simulink model "unicycle_nonlinear_Cl"  (R2024a)
settings: Solver=VariableStepAuto  StartTime=0.0  StopTime=30  RelTol=1e-3
values from neighbouring files (symbols this model uses):
  AK = AK2 - BK/(eye(p_y)-D22*DK)*D22*CK    [report_controller_output_feedback_Hinf.m]    (also in report_controller_output_feedback_LMI.m = A+L_gain*C2+B2*K_gain; report_controller_state_feedback_H2.m = zeros(n,n); report_controller_state_feedback_Hinf.m = zeros(n,n))
  BK = BK2*(eye(p_y)-D22*DK)    [report_controller_output_feedback_Hinf.m]    (also in report_controller_output_feedback_LMI.m = -L_gain; report_controller_state_feedback_H2.m = zeros(n,p_y); report_controller_state_feedback_Hinf.m = zeros(n,p_y))
  C2 = [1 0 0 0 ... (first row only)    [report_controller_output_feedback_Hinf.m]    (also in report_controller_output_feedback_LMI.m; report_controller_state_feedback_H2.m; report_controller_state_feedback_Hinf.m; report_model_negative_theta.m)
  CK = (eye(m)-DK*D22)*CK2    [report_controller_output_feedback_Hinf.m]    (also in report_controller_output_feedback_LMI.m = K_gain; report_controller_state_feedback_H2.m = zeros(m,n); report_controller_state_feedback_Hinf.m = zeros(m,n))
  DK = (eye(m)+DK2*D22)\DK2    [report_controller_output_feedback_Hinf.m]    (also in report_controller_output_feedback_LMI.m = zeros(m,p_y); report_controller_state_feedback_H2.m = K_gain; report_controller_state_feedback_Hinf.m = K_gain)
  equilibrium = asin((M_w+M_p)*R_w/(M_p*L)*sin(theta))-theta    [report_model_equilibrium.m]    (also in report_model_negative_theta.m = 0)
libraries: simulink x1
settings Model: Creator=Haven  LastModifiedBy=Haven

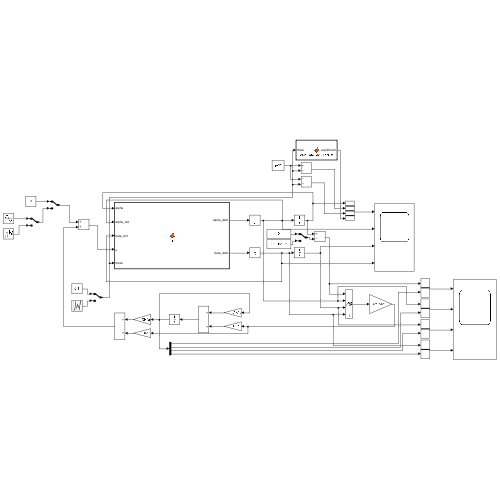
[thumbnail: Simulink's stored preview of the top-level diagram]
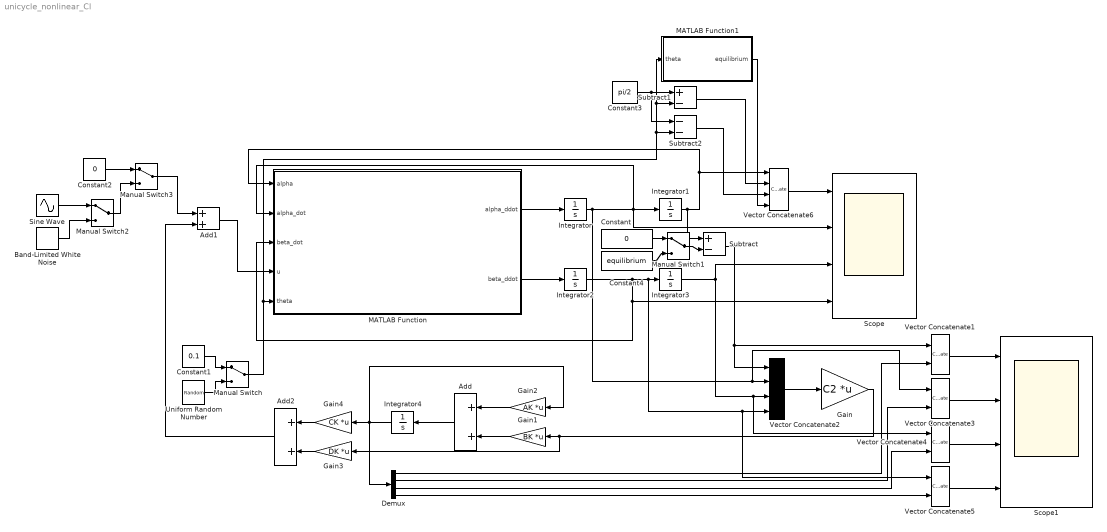
== system unicycle_nonlinear_Cl ==
  Add : Sum
  Add1 : Sum
  Add2 : Sum
  Band-Limited White Noise : simulink/Sources/Band-Limited White Noise  Cov=1  Ts=1  seed=[23341]
  Constant : Constant  Value=0
  Constant1 : Constant  Value=0.1
  Constant2 : Constant  Value=0
  Constant3 : Constant  Value=pi/2
  Constant4 : Constant  Value=equilibrium
  Demux : Demux
  Gain : Gain  Gain=C2  Multiplication=Matrix(K*u) (u vector)
  Gain1 : Gain  Gain=BK  Multiplication=Matrix(K*u)
  Gain2 : Gain  Gain=AK  Multiplication=Matrix(K*u)
  Gain3 : Gain  Gain=DK  Multiplication=Matrix(K*u)
  Gain4 : Gain  Gain=CK  Multiplication=Matrix(K*u)
  Integrator : Integrator  InitialCondition=-0.1
  Integrator1 : Integrator  InitialCondition=0.1
  Integrator2 : Integrator  InitialCondition=0.1
  Integrator3 : Integrator
  Integrator4 : Integrator
  MATLAB Function : MATLAB Function  TreatAsAtomicUnit=on
  MATLAB Function1 : MATLAB Function  TreatAsAtomicUnit=on
  Manual Switch{,1..3} (4 alike) : ManualSwitch
  Scope : Scope  NumInputPorts=4
  Scope1 : Scope  NumInputPorts=4
  Sine Wave : Sin  SampleTime=0
  Subtract : Sum  Inputs=+-
  Subtract1 : Sum  Inputs=+-
  Subtract2 : Sum  Inputs=--
  Uniform Random Number : UniformRandomNumber  Minimum=-0.1  Maximum=0.1  SampleTime=10
  Vector Concatenate{1,3..5} (4 alike) : Concatenate
  Vector Concatenate2 : Concatenate  NumInputs=4  Mode=Multidimensional array
  Vector Concatenate6 : Concatenate  NumInputs=4
  wires:
  MATLAB Function/1(alpha_ddot) -> Integrator/1
  Integrator1/1 -> Subtract/1, MATLAB Function/1(alpha), Vector Concatenate6/1
  Integrator/1 -> Scope/2, MATLAB Function/2(alpha_dot), Integrator1/1, Vector Concatenate3/1, Vector Concatenate2/2
  MATLAB Function/2(beta_ddot) -> Integrator2/1
  Integrator2/1 -> Vector Concatenate5/1, Vector Concatenate2/4, Integrator3/1, Scope/4, MATLAB Function/3(beta_dot)
  Integrator3/1 -> Vector Concatenate4/1, Vector Concatenate2/3, Scope/3
  Uniform Random Number/1 -> Manual Switch/2
  Constant1/1 -> Manual Switch/1
  Integrator4/1 -> Gain4/1, Gain2/1, Demux/1
  Manual Switch/1 -> Subtract2/2, Subtract1/2, MATLAB Function1/1(theta), MATLAB Function/5(theta)
  Vector Concatenate2/1 -> Gain/1
  Gain/1 -> Gain3/1, Gain1/1
  Vector Concatenate1/1 -> Scope1/1
  Vector Concatenate3/1 -> Scope1/2
  Vector Concatenate4/1 -> Scope1/3
  Vector Concatenate5/1 -> Scope1/4
  Demux/1 -> Vector Concatenate1/2
  Demux/2 -> Vector Concatenate3/2
  Demux/3 -> Vector Concatenate4/2
  Demux/4 -> Vector Concatenate5/2
  Sine Wave/1 -> Manual Switch2/1
  Manual Switch2/1 -> Manual Switch3/2
  Band-Limited White Noise/1 -> Manual Switch2/2
  Manual Switch3/1 -> Add1/1
  Constant2/1 -> Manual Switch3/1
  Add/1 -> Integrator4/1
  Gain2/1 -> Add/1
  Gain1/1 -> Add/2
  Gain3/1 -> Add2/2
  Add2/1 -> Add1/2
  Gain4/1 -> Add2/1
  Subtract/1 -> Vector Concatenate1/1, Vector Concatenate2/1
  Vector Concatenate6/1 -> Scope/1
  Constant3/1 -> Subtract2/1, Subtract1/1
  Subtract1/1 -> Vector Concatenate6/2
  Subtract2/1 -> Vector Concatenate6/3
  MATLAB Function1/1(equilibrium) -> Vector Concatenate6/4
  Add1/1 -> MATLAB Function/4(u)
  Manual Switch1/1 -> Subtract/2
  Constant/1 -> Manual Switch1/1
  Constant4/1 -> Manual Switch1/2

== matlab function unicycle_nonlinear_Cl/MATLAB Function1 ==
  data: theta input; equilibrium output
function equilibrium = calculate_equilibrium(theta)
g = 9.8;
M_p = 15.63;
M_w = 31.28;
R_w = 0.31;
L = 0.155;

equilibrium = asin((M_w+M_p)*R_w/(M_p*L)*sin(theta))-theta;

== matlab function unicycle_nonlinear_Cl/MATLAB Function ==
  data: alpha input; alpha_dot input; beta_dot input; u input; alpha_ddot output; theta input; beta_ddot output
function [alpha_ddot, beta_ddot] = fcn(alpha, alpha_dot, beta_dot,u,theta)
    g = 9.8;
    M_p = 15.63;
    M_w = 31.28;
    I_p = 3.55;
    I_w = 1.40;
    R_w = 0.31;
    L = 0.155;
    n = 19.56;
    k_T = 0.05;
    R = 1.2;
    k_e = 0.0534;
    
    tau = -(n^2 * k_T *k_e / R )* beta_dot + (n * k_T / R)*u;

    a = M_p* L^2 + I_p;
    b = M_p * R_w * L * cos(alpha+theta);
    d = M_w * R_w^2 + M_p * R_w^2 + I_w;

    c = -tau + M_p * L * g * sin(alpha + theta);
    e = tau - (M_p + M_w) * R_w * g * sin(theta) + alpha_dot^2 * M_p * R_w * L * sin(alpha + theta);

    alpha_ddot = (c*d - b*e)/(a*d - b*b);
    beta_ddot = (a*e - b*c)/(a*d - b*b);
end
